simulink model "MotorAndLed"  (R2013b)
settings: Solver=FixedStepDiscrete  StartTime=0.0  StopTime=30  FixedStep=0.1  RelTol=1e-3
libraries: ardrone_lib x3
settings Model: Creator=benjamin  LastModifiedBy=Jon Even ROSENGREN
settings OptimizationCC: InitFltsAndDblsToZero=on  OptimizeModelRefInitCode=on  LifeSpan=1
settings RTWCC: SystemTargetFile=ardrone.tlc  TemplateMakefile=ardrone.tmf  Description=AR.Drone_v2  ProcessScript=ardrone_make_rtw_hook  TargetLang=C++
settings CodeAppCC: IgnoreCustomStorageClasses=off
settings STFCustomTargetCC: GenerateSampleERTMain=on  ModelReferenceCompliant=off  CombineOutputUpdateFcns=on  ERTCustomFileBanners=on  SupportContinuousTime=off  SupportNonInlinedSFcns=off  MATLABClassNameForMDSCustomization=Simulink.SoftwareTarget.ERTCustomization  GRTInterface=off  SystemTargetFile=ardrone.tlc
settings ERTTargetCC: CodeReplacementLibrary=ANSI_C  GenerateSampleERTMain=on  ModelReferenceCompliant=off  ParMdlRefBuildCompliant=off  CompOptLevelCompliant=off  ConcurrentExecutionCompliant=off  ERTFirstTimeCompliant=off  ModelStepFunctionPrototypeControlCompliant=off  CPPClassGenCompliant=off  ERTSrcFileBannerTemplate=example_banner.tlc  ERTHdrFileBannerTemplate=example_banner.tlc  ERTCustomFileTemplate=ardrone_file_process.tlc

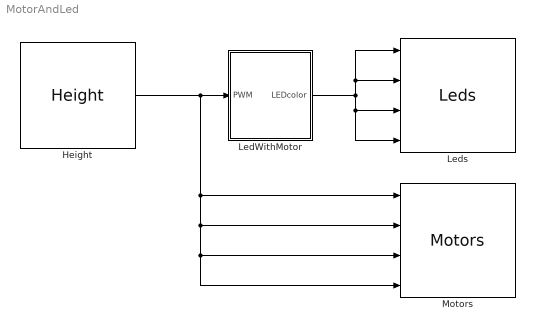
== system MotorAndLed ==
  Height : ardrone_lib/Height  SFunctionSpec=int16 y1 = Height_Get ()  ShowSpec=on
  LedWithMotor : Subsystem
  Leds : ardrone_lib/Leds  SystemSampleTime=-1
  Motors : ardrone_lib/Motors  SystemSampleTime=-1
  wires:
  Height/1 -> Motors/1, Motors/4, Motors/3, Motors/2, LedWithMotor/1(PWM)
  LedWithMotor/1(LEDcolor) -> Leds/4, Leds/3, Leds/2, Leds/1

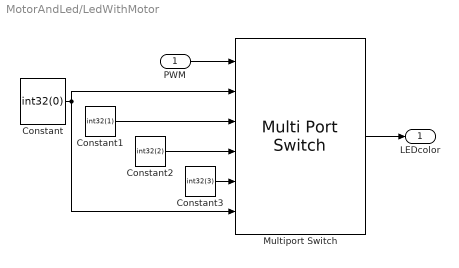
== system MotorAndLed/LedWithMotor ==
  PWM : Inport
  Constant : Constant  Value=int32(0)
  Constant1 : Constant  Value=int32(1)
  Constant2 : Constant  Value=int32(2)
  Constant3 : Constant  Value=int32(3)
  Multiport Switch : MultiPortSwitch  DataPortOrder=Specify indices  Inputs=4  DataPortIndices={[0.0:25.0],[26:50],[51:75],[76:100]}  DataPortForDefault=Additional data port  OutDataTypeStr=int32
  LEDcolor : Outport
  wires:
  Constant/1 -> Multiport Switch/2, Multiport Switch/6
  PWM/1 -> Multiport Switch/1
  Multiport Switch/1 -> LEDcolor/1
  Constant1/1 -> Multiport Switch/3
  Constant2/1 -> Multiport Switch/4
  Constant3/1 -> Multiport Switch/5
